simulink model "RadioReceiver_FP_clean_PIPELINED"  (R2017a)
settings: Solver=FixedStepDiscrete  StartTime=0.0  StopTime=10.0  RelTol=1e-3
InitFcn:
  | barker = comm.BarkerCode('SamplesPerFrame', 28, 'Length', 11);
  | seq = barker()+1;
  | M = 4;
  | hPSKModTrain   = comm.PSKModulator(M, ...
  |     'PhaseOffset',pi/4, ...
  |     'SymbolMapping','Binary');
  | xPreambleSeq = hPSKModTrain(seq);
  | 
  | 
  | %%%%%%%%%%%%
  | 
  | % AGC Preamble
  | reps = 5;
  | barker = comm.BarkerCode('SamplesPerFrame', 16, 'Length', 13);
  | seq = barker()+1;
  | %preamble = zeros(16*reps,1);
  | preambleFull = repmat(seq,reps,1);
  | rctFilt = comm.RaisedCosineTransmitFilter('FilterSpanInSymbols', 128,...
  | 'RolloffFactor',0.5,...
  | 'OutputSamplesPerSymbol',4);
  | preambleFullFilt = rctFilt(preambleFull);
  | 
  | %%%%%%%%%%%%
  | 
  | RadioSampleRate = 1e6;
  | %RadioSampleRate = 20e6;
  | RadioFrameLength = 1e5;
  | 
  | VibertiTracebackLength = 34+20;
  | numTrainingSamples = 250;
  | crc32Poly = [1 0 0 0 0 0 1 0 0 1 1 0 0 0 0 0 1 0 0 0 1 1 1 0 1 1 0 1 1 0 1 1 1];
  | crcDecodeLag = length(crc32Poly)-1+2;
  | 
  | %%%%%%%%%%%%
  | 
  | beta = 0.5;
  | span = 8;
  | sps = 4;
  | filterGain = 1;
  | coeff = rcosdesign(beta, span, sps, 'sqrt')*filterGain;
  | 
  | %%%%%%%%%%%%
  | 
  | samplesPerSymbol = 4;
  | maxPacketBits = 8*1500;
  | bItsPerSymbol = 2;
  | CodeRate = 2;
  | tailSymbols = 40;
  | maxPayloadSymbols = maxPacketBits*CodeRate/bItsPerSymbol+tailSymbols;
undefined symbols (not defined in the file or in its folder): j
libraries: dsphdlfiltering x20, simulink x11, dspstat3 x2, commdigbbndpm3 x2, commsource2 x1, commcrc2 x1, commcnvcod2 x1, commseqgen3 x1, commutil2 x1, hdlsllib x1
(part 1 of 2)
settings Model: DataTypeOverride=Off  MinMaxOverflowLogging=MinMaxAndOverflow  FPTRunName=NoOverride  Creator=tcollins  LastModifiedBy=tcollins
settings DataIOCC: SaveOutput=off  SaveTime=off
settings OptimizationCC: BlockReduction=off  ConditionallyExecuteInputs=off  DefaultParameterBehavior=Inlined
settings DebuggingCC: AlgebraicLoopMsg=error  SingleTaskRateTransMsg=error
settings HardwareCC: ProdBitPerPointer=32  ProdBitPerSizeT=32  ProdBitPerPtrDiffT=32  ProdLargestAtomicFloat=None  ProdIntDivRoundTo=Undefined  ProdEndianess=Unspecified  ProdWordSize=32  ProdHWDeviceType=ASIC/FPGA->ASIC/FPGA  ProdEqTarget=off

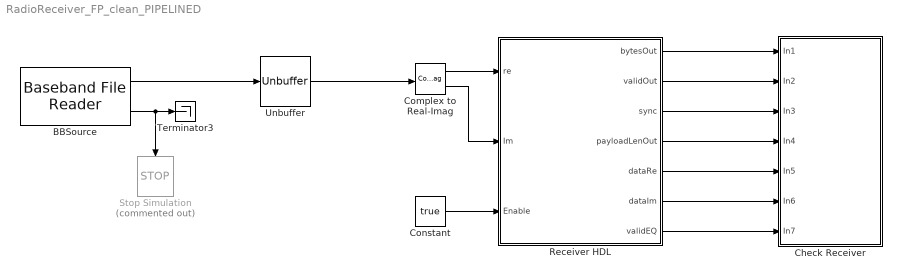
== system RadioReceiver_FP_clean_PIPELINED ==
  BBSource : commsource2/Baseband File Reader  Filename=/home/tcollins/currentWork/modem-phy/FixedPoint/Pluto3.bb  InheritSampleTimeFromFile=off  SampleTime=100000/(RadioSampleRate)  SamplesPerFrame=100000  CyclicRepetition=off  FileEndOutputPort=on  SimulateUsing=Interpreted execution
      settings: SourceProductName=Communications System Toolbox  SourceProductBaseCode=CM
  Check Receiver : Subsystem
  Complex to Real-Imag : ComplexToRealImag
  Constant : Constant  Value=true  SampleTime=1/RadioSampleRate
  Receiver HDL : Subsystem  TreatAsAtomicUnit=on
  Stop Simulation : Stop  Commented=on
  Terminator3 : Terminator
  Unbuffer : Unbuffer
  wires:
  BBSource/1 -> Unbuffer/1
  Constant/1 -> Receiver HDL/3(Enable)
  Complex to Real-Imag/1 -> Receiver HDL/1(re)
  Complex to Real-Imag/2 -> Receiver HDL/2(Im)
  BBSource/2 -> Stop Simulation/1, Terminator3/1
  Unbuffer/1 -> Complex to Real-Imag/1
  Receiver HDL/1(bytesOut) -> Check Receiver/1(In1)
  Receiver HDL/2(validOut) -> Check Receiver/2(In2)
  Receiver HDL/3(sync) -> Check Receiver/3(In3)
  Receiver HDL/4(payloadLenOut) -> Check Receiver/4(In4)
  Receiver HDL/5(dataRe) -> Check Receiver/5(In5)
  Receiver HDL/6(dataIm) -> Check Receiver/6(In6)
  Receiver HDL/7(validEQ) -> Check Receiver/7(In7)

== system RadioReceiver_FP_clean_PIPELINED/Check Receiver ==
  In1 : Inport
  In2 : Inport  Port=2
  In3 : Inport  Port=3
  In4 : Inport  Port=4
  In5 : Inport  Port=5
  In6 : Inport  Port=6
  In7 : Inport  Port=7
  Constellation Diagram : Subsystem
  DMA Capture : MATLAB Function  TreatAsAtomicUnit=on
  Real-Imag to Complex : RealImagToComplex
  wires:
  Real-Imag to Complex/1 -> Constellation Diagram/1(In1)
  In5/1 -> Real-Imag to Complex/1
  In3/1 -> DMA Capture/3(sync)
  In7/1 -> Constellation Diagram/Enable
  In2/1 -> DMA Capture/2(validOut)
  In1/1 -> DMA Capture/1(bytes)
  In4/1 -> DMA Capture/4(payloadLen)
  In6/1 -> Real-Imag to Complex/2

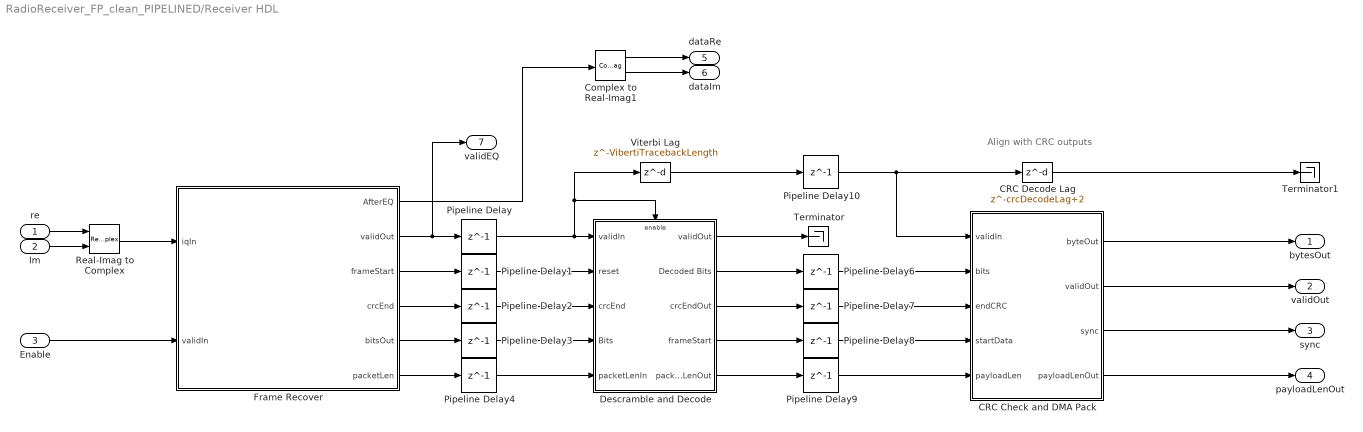
== system RadioReceiver_FP_clean_PIPELINED/Receiver HDL ==
  note: Align with CRC outputs
  re : Inport  OutDataTypeStr=int16
  Im : Inport  Port=2  OutDataTypeStr=int16
  Enable : Inport  Port=3
  CRC Check and DMA Pack : Subsystem
  CRC Decode Lag : Delay  DelayLength=crcDecodeLag+2
  Complex to Real-Imag1 : ComplexToRealImag
  Descramble and Decode : Subsystem  TreatAsAtomicUnit=on
  Frame Recover : Subsystem
  Pipeline Delay{,1..4,6..10} (10 alike) : Delay  DelayLength=1
  Real-Imag to Complex : RealImagToComplex
  Terminator : Terminator
  Terminator1 : Terminator
  Viterbi Lag : Delay  DelayLength=VibertiTracebackLength
  bytesOut : Outport
  validOut : Outport  Port=2
  sync : Outport  Port=3
  payloadLenOut : Outport  Port=4
  dataRe : Outport  Port=5
  dataIm : Outport  Port=6
  validEQ : Outport  Port=7
  wires:
  re/1 -> Real-Imag to Complex/1
  Im/1 -> Real-Imag to Complex/2
  Complex to Real-Imag1/2 -> dataIm/1
  Complex to Real-Imag1/1 -> dataRe/1
  Frame Recover/6(packetLen) -> Pipeline Delay4/1
  Frame Recover/2(validOut) -> validEQ/1, Pipeline Delay/1
  Real-Imag to Complex/1 -> Frame Recover/1(iqIn)
  Enable/1 -> Frame Recover/2(validIn)
  Frame Recover/1(AfterEQ) -> Complex to Real-Imag1/1
  Frame Recover/3(frameStart) -> Pipeline Delay1/1
  Frame Recover/4(crcEnd) -> Pipeline Delay2/1
  Frame Recover/5(bitsOut) -> Pipeline Delay3/1
  Descramble and Decode/3(crcEndOut) -> Pipeline Delay7/1
  Descramble and Decode/4(frameStart) -> Pipeline Delay8/1
  Descramble and Decode/5(packetLenOut) -> Pipeline Delay9/1
  CRC Check and DMA Pack/1(byteOut) -> bytesOut/1
  CRC Check and DMA Pack/2(validOut) -> validOut/1
  Pipeline Delay1/1 -> Descramble and Decode/2(reset)
  Pipeline Delay3/1 -> Descramble and Decode/4(Bits)
  Pipeline Delay4/1 -> Descramble and Decode/5(packetLenIn)
  Pipeline Delay8/1 -> CRC Check and DMA Pack/4(startData)
  Pipeline Delay6/1 -> CRC Check and DMA Pack/2(bits)
  Pipeline Delay9/1 -> CRC Check and DMA Pack/5(payloadLen)
  Pipeline Delay7/1 -> CRC Check and DMA Pack/3(endCRC)
  CRC Check and DMA Pack/3(sync) -> sync/1
  Pipeline Delay2/1 -> Descramble and Decode/3(crcEnd)
  Descramble and Decode/2(Decoded Bits) -> Pipeline Delay6/1
  Pipeline Delay10/1 -> CRC Check and DMA Pack/1(validIn), CRC Decode Lag/1
  CRC Check and DMA Pack/4(payloadLenOut) -> payloadLenOut/1
  Pipeline Delay/1 -> Descramble and Decode/Enable, Viterbi Lag/1, Descramble and Decode/1(validIn)
  Descramble and Decode/1(validOut) -> Terminator/1
  Viterbi Lag/1 -> Pipeline Delay10/1
  CRC Decode Lag/1 -> Terminator1/1

== system RadioReceiver_FP_clean_PIPELINED/Check Receiver/Constellation Diagram ==
  In1 : Inport
  Enable : EnablePort
  After EQ (Outside) : ConstellationDiagram
  wires:
  In1/1 -> After EQ (Outside)/1

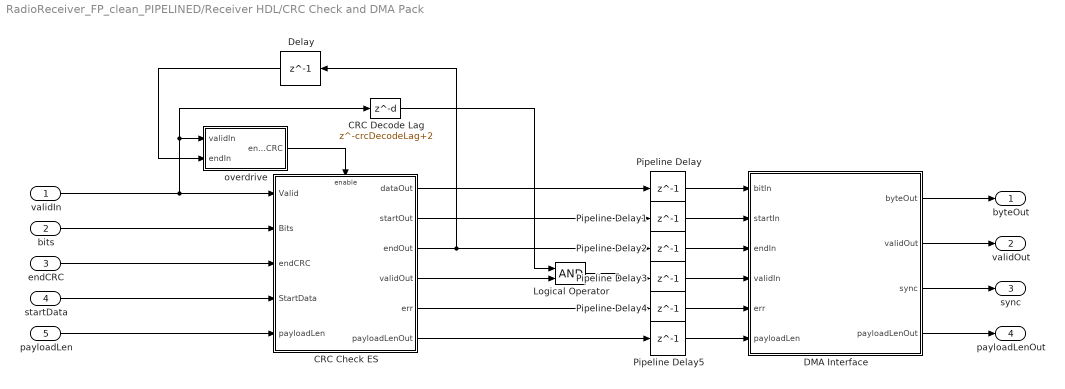
== system RadioReceiver_FP_clean_PIPELINED/Receiver HDL/CRC Check and DMA Pack ==
  validIn : Inport
  bits : Inport  Port=2
  endCRC : Inport  Port=3
  startData : Inport  Port=4
  payloadLen : Inport  Port=5
  CRC Check ES : Subsystem
  CRC Decode Lag : Delay  DelayLength=crcDecodeLag+2
  DMA Interface : Subsystem
  Delay : Delay  DelayLength=1
  Logical Operator : Logic  AllPortsSameDT=off  OutDataTypeStr=boolean
  Pipeline Delay{,1..5} (6 alike) : Delay  DelayLength=1
  overdrive : MATLAB Function  TreatAsAtomicUnit=on
  byteOut : Outport
  validOut : Outport  Port=2
  sync : Outport  Port=3
  payloadLenOut : Outport  Port=4
  wires:
  DMA Interface/2(validOut) -> validOut/1
  CRC Check ES/3(endOut) -> Delay/1, Pipeline Delay2/1
  DMA Interface/1(byteOut) -> byteOut/1
  CRC Check ES/2(startOut) -> Pipeline Delay1/1
  CRC Check ES/1(dataOut) -> Pipeline Delay/1
  CRC Check ES/5(err) -> Pipeline Delay4/1
  bits/1 -> CRC Check ES/2(Bits)
  DMA Interface/3(sync) -> sync/1
  payloadLen/1 -> CRC Check ES/5(payloadLen)
  startData/1 -> CRC Check ES/4(StartData)
  CRC Check ES/6(payloadLenOut) -> Pipeline Delay5/1
  endCRC/1 -> CRC Check ES/3(endCRC)
  Pipeline Delay/1 -> DMA Interface/1(bitIn)
  Pipeline Delay1/1 -> DMA Interface/2(startIn)
  Pipeline Delay2/1 -> DMA Interface/3(endIn)
  Pipeline Delay3/1 -> DMA Interface/4(validIn)
  Pipeline Delay4/1 -> DMA Interface/5(err)
  Pipeline Delay5/1 -> DMA Interface/6(payloadLen)
  CRC Decode Lag/1 -> Logical Operator/1
  CRC Check ES/4(validOut) -> Logical Operator/2
  validIn/1 -> CRC Check ES/1(Valid), CRC Decode Lag/1, overdrive/1(validIn)
  Delay/1 -> overdrive/2(endIn)
  DMA Interface/4(payloadLenOut) -> payloadLenOut/1
  Logical Operator/1 -> Pipeline Delay3/1
  overdrive/1(enableCRC) -> CRC Check ES/Enable

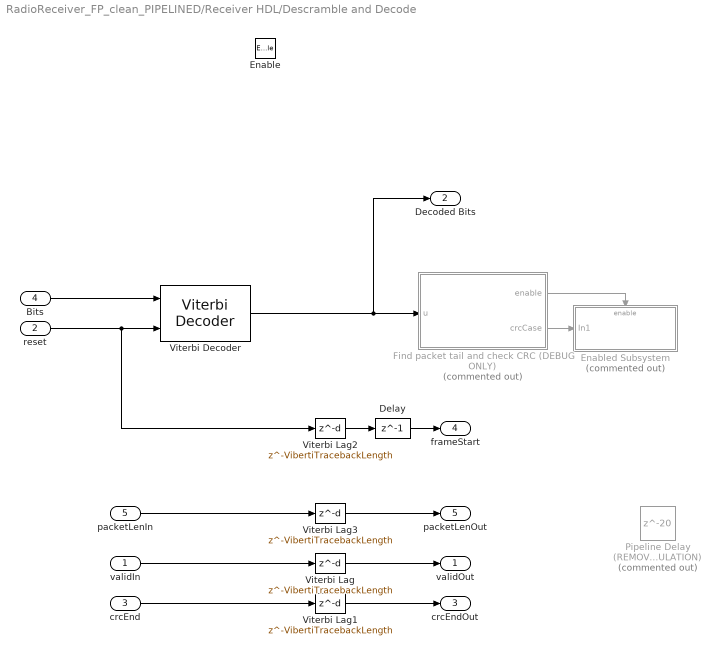
== system RadioReceiver_FP_clean_PIPELINED/Receiver HDL/Descramble and Decode ==
  validIn : Inport
  reset : Inport  Port=2
  crcEnd : Inport  Port=3
  Bits : Inport  Port=4
  packetLenIn : Inport  Port=5
  Enable : EnablePort
  Delay : Delay  DelayLength=1
  Enabled Subsystem : Subsystem  Commented=on  TreatAsAtomicUnit=on
  Find packet tail and check CRC (DEBUG ONLY) : MATLAB Function  Commented=on  TreatAsAtomicUnit=on
  "Pipeline Delay (REMOVE BEFORE SYNTH, ONLY FOR SIMULATION)" : Delay  Commented=on  DelayLength=20
  Viterbi Decoder : commcnvcod2/Viterbi Decoder  trellis=poly2trellis(7, [171 133])  isPunctured=off  punctureVector=[1; 1; 0; 1; 0; 1]  erasures=off  dectype=Hard decision  nsdecb=4  runSigValErrCheck=off  tbdepth=VibertiTracebackLength-20  opmode=Continuous  reset=on  delayedResetAction=on  smWordLength=16  outDataType=boolean
      settings: SourceProductName=Communications System Toolbox  SourceProductBaseCode=CM
  Viterbi Lag{,1..3} (4 alike) : Delay  DelayLength=VibertiTracebackLength
  validOut : Outport  InitialOutput=0
  Decoded Bits : Outport  Port=2  InitialOutput=0
  crcEndOut : Outport  Port=3  InitialOutput=0
  frameStart : Outport  Port=4  InitialOutput=0
  packetLenOut : Outport  Port=5  InitialOutput=0
  wires:
  reset/1 -> Viterbi Lag2/1, Viterbi Decoder/2
  Find packet tail and check CRC (DEBUG ONLY)/1(enable) -> Enabled Subsystem/Enable
  Find packet tail and check CRC (DEBUG ONLY)/2(crcCase) -> Enabled Subsystem/1(In1)
  Bits/1 -> Viterbi Decoder/1
  validIn/1 -> Viterbi Lag/1
  Viterbi Lag3/1 -> packetLenOut/1
  Viterbi Lag2/1 -> Delay/1
  Viterbi Lag1/1 -> crcEndOut/1
  Viterbi Lag/1 -> validOut/1
  packetLenIn/1 -> Viterbi Lag3/1
  crcEnd/1 -> Viterbi Lag1/1
  Delay/1 -> frameStart/1
  Viterbi Decoder/1 -> Decoded Bits/1, Find packet tail and check CRC (DEBUG ONLY)/1(u)

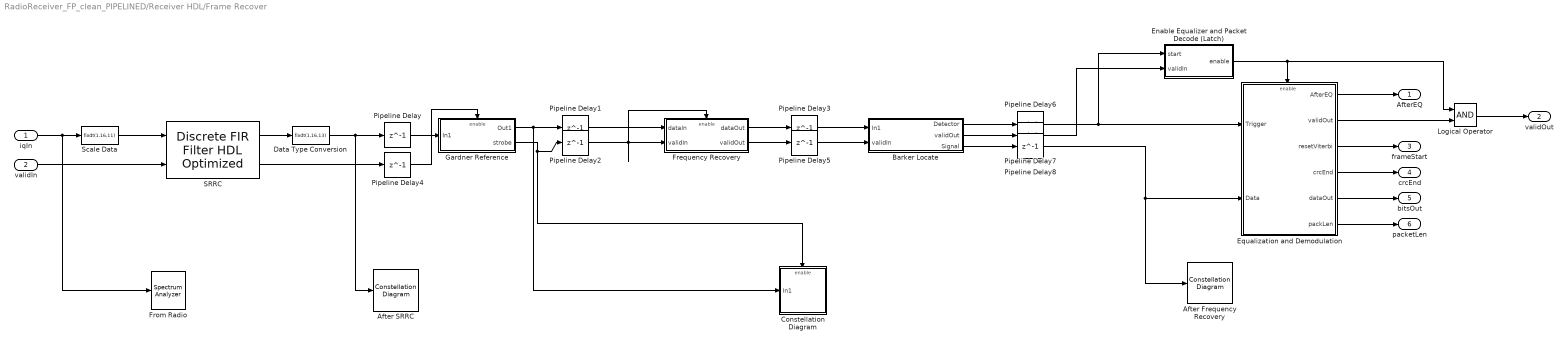
== system RadioReceiver_FP_clean_PIPELINED/Receiver HDL/Frame Recover ==
  iqIn : Inport
  validIn : Inport  Port=2
  After Frequency Recovery : ConstellationDiagram
  After SRRC : ConstellationDiagram
  Barker Locate : Subsystem  mask{Threshold=1}
  Constellation Diagram : Subsystem
  Data Type Conversion : DataTypeConversion  OutDataTypeStr=fixdt(1,16,13)
  Enable Equalizer and Packet Decode (Latch) : MATLAB Function  TreatAsAtomicUnit=on
  Equalization and Demodulation : Subsystem
  Frequency Recovery : Subsystem
  From Radio : SpectrumAnalyzer
  Gardner Reference : Subsystem
  Logical Operator : Logic  AllPortsSameDT=off  OutDataTypeStr=boolean
  Pipeline Delay{,1..8} (9 alike) : Delay  DelayLength=1
  SRRC : dsphdlfiltering/Discrete FIR Filter HDL Optimized  Numerator=coeff  Sharing=off  SharingFactor=2  SimulateUsing=Code generation  roundingMode=Floor  overflowMode=on  CoefficientsDataTypeStr=Inherit: Same word length as input  CoefficientsMin=[]  CoefficientsMax=[]  OutputDataTypeStr=fixdt(1,16,11)  OutputMin=[]  OutputMax=[]  ValidInPort=on  ReadyPort=off
      settings: SourceProductName=DSP System Toolbox  SourceProductBaseCode=DS
  Scale Data : DataTypeConversion  OutDataTypeStr=fixdt(1,16,11)  ConvertRealWorld=Stored Integer (SI)  SaturateOnIntegerOverflow=on
  AfterEQ : Outport
  validOut : Outport  Port=2
  frameStart : Outport  Port=3
  crcEnd : Outport  Port=4
  bitsOut : Outport  Port=5
  packetLen : Outport  Port=6
  wires:
  Equalization and Demodulation/3(resetViterbi) -> frameStart/1
  Barker Locate/2(validOut) -> Pipeline Delay7/1
  Equalization and Demodulation/4(crcEnd) -> crcEnd/1
  Frequency Recovery/2(validOut) -> Pipeline Delay5/1
  Enable Equalizer and Packet Decode (Latch)/1(enable) -> Logical Operator/1, Equalization and Demodulation/Enable
  Equalization and Demodulation/5(dataOut) -> bitsOut/1
  SRRC/2 -> Pipeline Delay4/1
  SRRC/1 -> Data Type Conversion/1
  iqIn/1 -> From Radio/1, Scale Data/1
  validIn/1 -> SRRC/2
  Barker Locate/3(Signal) -> Pipeline Delay8/1
  Frequency Recovery/1(dataOut) -> Pipeline Delay3/1
  Equalization and Demodulation/2(validOut) -> Logical Operator/2
  Scale Data/1 -> SRRC/1
  Equalization and Demodulation/6(packLen) -> packetLen/1
  Barker Locate/1(Detector) -> Pipeline Delay6/1
  Equalization and Demodulation/1(AfterEQ) -> AfterEQ/1
  Pipeline Delay1/1 -> Frequency Recovery/1(dataIn)
  Pipeline Delay2/1 -> Frequency Recovery/Enable, Frequency Recovery/2(validIn)
  Pipeline Delay3/1 -> Barker Locate/1(In1)
  Pipeline Delay5/1 -> Barker Locate/2(validIn)
  Pipeline Delay6/1 -> Enable Equalizer and Packet Decode (Latch)/1(start), Equalization and Demodulation/1(Trigger)
  Pipeline Delay7/1 -> Enable Equalizer and Packet Decode (Latch)/2(validIn)
  Pipeline Delay8/1 -> Equalization and Demodulation/2(Data), After Frequency Recovery/1
  Logical Operator/1 -> validOut/1
  Data Type Conversion/1 -> After SRRC/1, Pipeline Delay/1
  Pipeline Delay/1 -> Gardner Reference/1(In1)
  Gardner Reference/2(strobe) -> Pipeline Delay2/1, Constellation Diagram/Enable
  Gardner Reference/1(Out1) -> Constellation Diagram/1(In1), Pipeline Delay1/1
  Pipeline Delay4/1 -> Gardner Reference/Enable

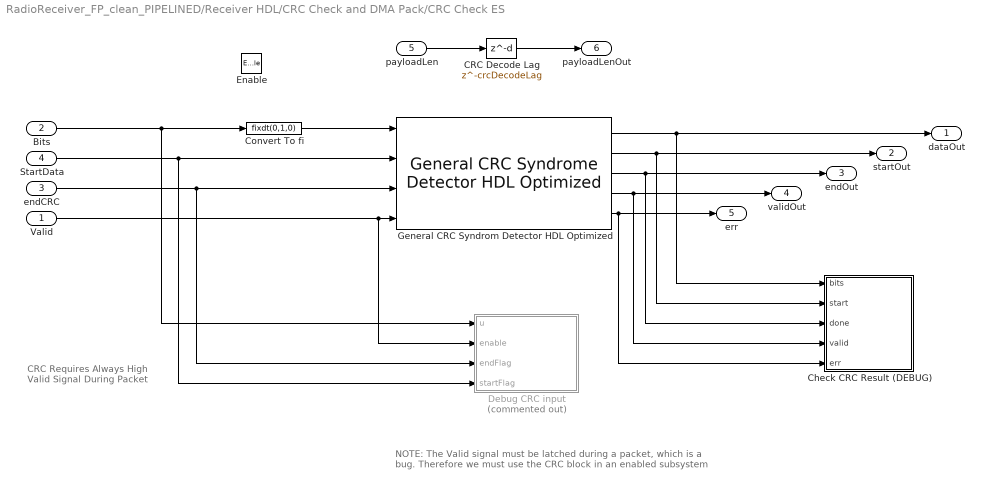
== system RadioReceiver_FP_clean_PIPELINED/Receiver HDL/CRC Check and DMA Pack/CRC Check ES ==
  note: NOTE:
      | 	The Valid signal must be latched during a packet, which is
      | 	a bug.  Therefore we must use the CRC block in an enabled
      | 	subsystem
  note: CRC Requires
      | Always High
      | Valid Signal During
      | Packet
  Valid : Inport
  Bits : Inport  Port=2
  endCRC : Inport  Port=3
  StartData : Inport  Port=4
  payloadLen : Inport  Port=5
  Enable : EnablePort
  CRC Decode Lag : Delay  DelayLength=crcDecodeLag
  Check CRC Result (DEBUG) : MATLAB Function  TreatAsAtomicUnit=on
  Convert To fi : DataTypeConversion  OutDataTypeStr=fixdt(0,1,0)  SaturateOnIntegerOverflow=on
  Debug CRC input : MATLAB Function  Commented=on  TreatAsAtomicUnit=on
  General CRC Syndrom Detector HDL Optimized : commcrc2/General CRC Syndrome Detector HDL Optimized  Polynomial=crc32Poly  InitialState=0  DirectMethod=off  ReflectInput=off  ReflectCRCChecksum=off  FinalXORValue=0  SimulateUsing=Code generation
      settings: SourceProductName=Communications System Toolbox  SourceProductBaseCode=CM
  dataOut : Outport  InitialOutput=0
  startOut : Outport  Port=2  InitialOutput=0
  endOut : Outport  Port=3  InitialOutput=0
  validOut : Outport  Port=4  InitialOutput=0
  err : Outport  Port=5  InitialOutput=0
  payloadLenOut : Outport  Port=6  InitialOutput=0
  wires:
  Bits/1 -> Convert To fi/1, Debug CRC input/1(u)
  General CRC Syndrom Detector HDL Optimized/1 -> Check CRC Result (DEBUG)/1(bits), dataOut/1
  General CRC Syndrom Detector HDL Optimized/3 -> Check CRC Result (DEBUG)/3(done), endOut/1
  General CRC Syndrom Detector HDL Optimized/4 -> Check CRC Result (DEBUG)/4(valid), validOut/1
  General CRC Syndrom Detector HDL Optimized/5 -> Check CRC Result (DEBUG)/5(err), err/1
  General CRC Syndrom Detector HDL Optimized/2 -> Check CRC Result (DEBUG)/2(start), startOut/1
  Convert To fi/1 -> General CRC Syndrom Detector HDL Optimized/1
  payloadLen/1 -> CRC Decode Lag/1
  CRC Decode Lag/1 -> payloadLenOut/1
  StartData/1 -> Debug CRC input/4(startFlag), General CRC Syndrom Detector HDL Optimized/2
  endCRC/1 -> Debug CRC input/3(endFlag), General CRC Syndrom Detector HDL Optimized/3
  Valid/1 -> Debug CRC input/2(enable), General CRC Syndrom Detector HDL Optimized/4

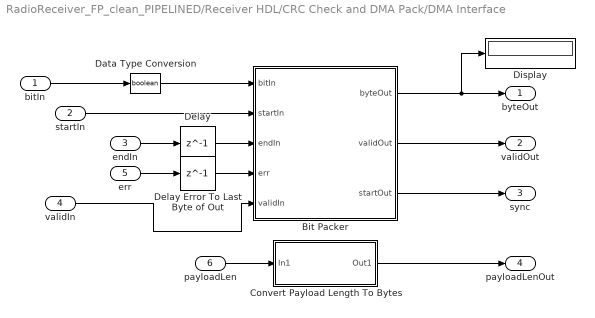
== system RadioReceiver_FP_clean_PIPELINED/Receiver HDL/CRC Check and DMA Pack/DMA Interface ==
  bitIn : Inport
  startIn : Inport  Port=2
  endIn : Inport  Port=3
  validIn : Inport  Port=4
  err : Inport  Port=5
  payloadLen : Inport  Port=6
  Bit Packer : MATLAB Function  TreatAsAtomicUnit=on
  Convert Payload Length To Bytes : Subsystem
  Data Type Conversion : DataTypeConversion  OutDataTypeStr=boolean
  Delay : Delay  DelayLength=1
  Delay Error To Last Byte of Out : Delay  DelayLength=1
  Display : Display
  byteOut : Outport
  validOut : Outport  Port=2
  sync : Outport  Port=3
  payloadLenOut : Outport  Port=4
  wires:
  bitIn/1 -> Data Type Conversion/1
  Delay/1 -> Bit Packer/3(endIn)
  Delay Error To Last Byte of Out/1 -> Bit Packer/4(err)
  Bit Packer/2(validOut) -> validOut/1
  Bit Packer/3(startOut) -> sync/1
  Bit Packer/1(byteOut) -> Display/1, byteOut/1
  err/1 -> Delay Error To Last Byte of Out/1
  validIn/1 -> Bit Packer/5(validIn)
  endIn/1 -> Delay/1
  startIn/1 -> Bit Packer/2(startIn)
  Data Type Conversion/1 -> Bit Packer/1(bitIn)
  payloadLen/1 -> Convert Payload Length To Bytes/1(In1)
  Convert Payload Length To Bytes/1(Out1) -> payloadLenOut/1

== system RadioReceiver_FP_clean_PIPELINED/Receiver HDL/Descramble and Decode/Enabled Subsystem ==
  In1 : Inport
  Enable : EnablePort
  To Workspace : ToWorkspace  VariableName=crcConditions  SaveFormat=Structure  SampleTime=-1
  wires:
  In1/1 -> To Workspace/1

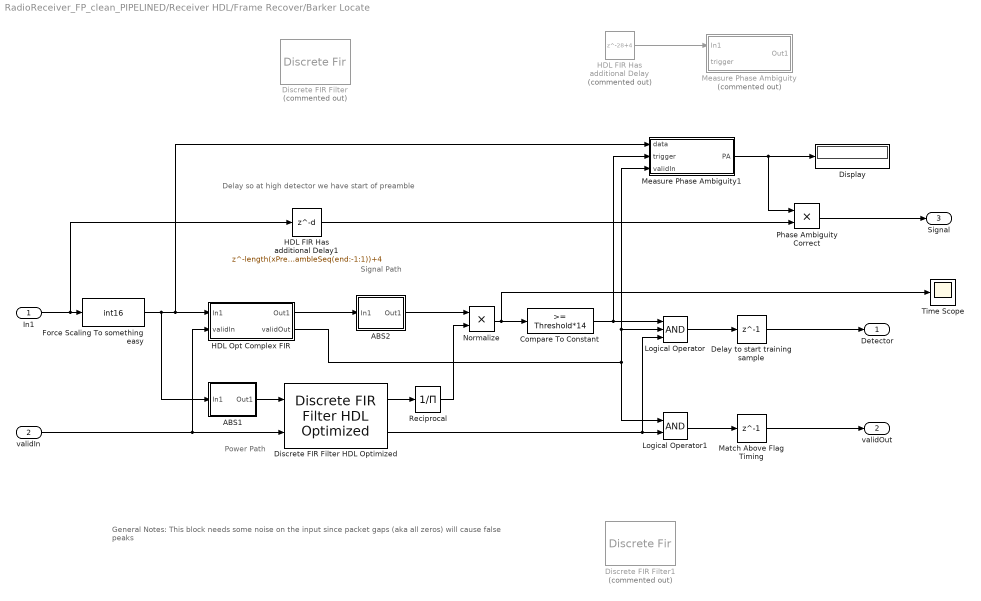
== system RadioReceiver_FP_clean_PIPELINED/Receiver HDL/Frame Recover/Barker Locate ==
  note: General Notes:
      | This block needs some noise on the input since packet gaps (aka all zeros) will cause false peaks
  note: Delay so at high detector we have start of preamble
  note: Power Path
  note: Signal Path
  In1 : Inport
  validIn : Inport  Port=2
  ABS1 : Subsystem
  ABS2 : Subsystem
  Compare To Constant : simulink/Logic and Bit Operations/Compare To Constant  relop=>=  const=Threshold*14  OutDataTypeStr=boolean
  "Delay to start training sample " : Delay  DelayLength=1
  Discrete FIR Filter : DiscreteFir  Commented=on  Coefficients=xPreambleSeq(end:-1:1).'  AccumDataTypeStr=Inherit: Same as product output  OutDataTypeStr=int16
  Discrete FIR Filter HDL Optimized : dsphdlfiltering/Discrete FIR Filter HDL Optimized  Numerator=ones(1,length(xPreambleSeq)*1)/1  Sharing=off  SharingFactor=2  SimulateUsing=Code generation  roundingMode=Floor  overflowMode=off  CoefficientsDataTypeStr=Inherit: Same word length as input  CoefficientsMin=[]  CoefficientsMax=[]  OutputDataTypeStr=fixdt(1,17,0)  OutputMin=[]  OutputMax=[]  ValidInPort=on  ReadyPort=off
      settings: SourceProductName=DSP System Toolbox  SourceProductBaseCode=DS
  Discrete FIR Filter1 : DiscreteFir  Commented=on  Coefficients=ones(1,length(xPreambleSeq)*1)/1  AccumDataTypeStr=Inherit: Same as product output  OutDataTypeStr=int16  SaturateOnIntegerOverflow=on
  Display : Display
  Force Scaling To something easy : DataTypeConversion  OutDataTypeStr=int16  SaturateOnIntegerOverflow=on
  HDL FIR Has additional Delay : Delay  Commented=on  DelayLength=28+4
  HDL FIR Has additional Delay1 : Delay  DelayLength=length(xPreambleSeq(end:-1:1))+4
  HDL Opt Complex FIR : Subsystem  mask{Taps=xPreambleSeq(end:-1:1).'}
  Logical Operator : Logic  Inputs=3  AllPortsSameDT=off  OutDataTypeStr=boolean
  Logical Operator1 : Logic  AllPortsSameDT=off  OutDataTypeStr=boolean
  Match Above Flag Timing : Delay  DelayLength=1
  Measure Phase Ambiguity : Subsystem  Commented=on
  Measure Phase Ambiguity1 : Subsystem
  Normalize : Product  Inputs=**  OutDataTypeStr=int16  RndMeth=Simplest  SaturateOnIntegerOverflow=on
  Phase Ambiguity Correct : Product  OutDataTypeStr=fixdt(1,16,14)
  Reciprocal : Product  Inputs=/  SaturateOnIntegerOverflow=on  RndMeth=Zero
  Time Scope : Scope
  Detector : Outport
  validOut : Outport  Port=2
  Signal : Outport  Port=3
  wires:
  HDL Opt Complex FIR/1(Out1) -> ABS2/1(In1)
  ABS2/1(Out1) -> Normalize/1
  "Delay to start training sample "/1 -> Detector/1
  Normalize/1 -> Time Scope/1, Compare To Constant/1
  In1/1 -> HDL FIR Has additional Delay1/1, Force Scaling To something easy/1
  ABS1/1(Out1) -> Discrete FIR Filter HDL Optimized/1
  Logical Operator/1 -> "Delay to start training sample "/1
  Logical Operator1/1 -> Match Above Flag Timing/1
  Measure Phase Ambiguity1/1(PA) -> Display/1, Phase Ambiguity Correct/1
  validIn/1 -> HDL Opt Complex FIR/2(validIn), Discrete FIR Filter HDL Optimized/2
  Discrete FIR Filter HDL Optimized/2 -> Logical Operator1/2, Logical Operator/3
  HDL Opt Complex FIR/2(validOut) -> Logical Operator1/1, Measure Phase Ambiguity1/3(validIn), Logical Operator/2
  Phase Ambiguity Correct/1 -> Signal/1
  HDL FIR Has additional Delay1/1 -> Phase Ambiguity Correct/2
  Force Scaling To something easy/1 -> ABS1/1(In1), HDL Opt Complex FIR/1(In1), Measure Phase Ambiguity1/1(data)
  Compare To Constant/1 -> Measure Phase Ambiguity1/2(trigger), Logical Operator/1
  HDL FIR Has additional Delay/1 -> Measure Phase Ambiguity/1(In1)
  Discrete FIR Filter HDL Optimized/1 -> Reciprocal/1
  Reciprocal/1 -> Normalize/2
  Match Above Flag Timing/1 -> validOut/1

== system RadioReceiver_FP_clean_PIPELINED/Receiver HDL/Frame Recover/Constellation Diagram ==
  In1 : Inport
  Enable : EnablePort
  After Timing Recovery : ConstellationDiagram
  wires:
  In1/1 -> After Timing Recovery/1

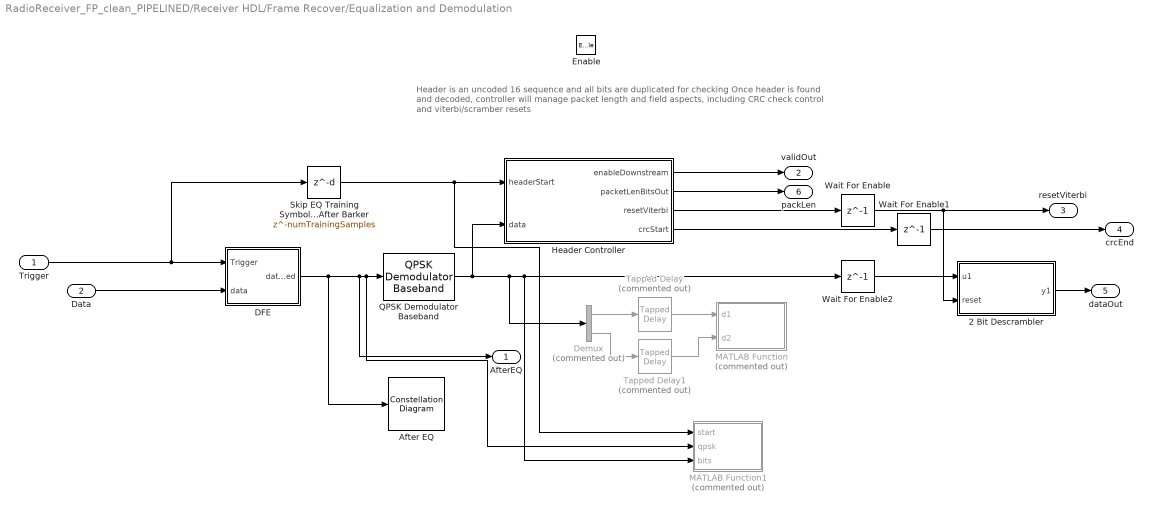
== system RadioReceiver_FP_clean_PIPELINED/Receiver HDL/Frame Recover/Equalization and Demodulation ==
  note: Header is an uncoded 16 sequence and all bits are duplicated for checking
      |
      | Once header is found and decoded, controller will manage packet length and field aspects,
      | including CRC check control and viterbi/scramber resets
  Trigger : Inport
  Data : Inport  Port=2
  Enable : EnablePort
  2 Bit Descrambler : Subsystem  mask{polynom=[1 1 0 1 0 1 0 1], initstate=[0 1 0 0 0 1 0]}
      mask prompts: polynom "Polynomial"; initstate "Inital State"
      mask Display: fprintf('HDL Descrambler')
  After EQ : ConstellationDiagram
  DFE : Subsystem
  Demux : Demux  Commented=on  Outputs=2
  Header Controller : MATLAB Function  TreatAsAtomicUnit=on
  MATLAB Function : MATLAB Function  Commented=on  TreatAsAtomicUnit=on
  MATLAB Function1 : MATLAB Function  Commented=on  TreatAsAtomicUnit=on
  QPSK Demodulator Baseband : commdigbbndpm3/QPSK Demodulator Baseband  OutType=Bit  DecType=Hard decision  VarSource=Dialog  Variance=1  Dec=Binary  Ph=pi/4  outDtype1=boolean  outDtype2=Inherit via internal rule  derotateFactorWordLen=16  derotateFactorDataTypeStr=Inherit: Same word length as input  derotateFactorLastDataTypeStr=Inherit: Same word length as input
  Skip EQ Training Symbols After Barker : Delay  DelayLength=numTrainingSamples
  Tapped Delay : simulink/Discrete/Tapped Delay  Commented=on  vinit=0.0  samptime=-1  NumDelays=16  DelayOrder=Oldest  includeCurrent=off
  Tapped Delay1 : simulink/Discrete/Tapped Delay  Commented=on  vinit=0.0  samptime=-1  NumDelays=16  DelayOrder=Oldest  includeCurrent=off
  Wait For Enable : Delay  DelayLength=1
  Wait For Enable1 : Delay  DelayLength=1
  Wait For Enable2 : Delay  DelayLength=1
  AfterEQ : Outport  InitialOutput=0
  validOut : Outport  Port=2  InitialOutput=0
  resetViterbi : Outport  Port=3  InitialOutput=0
  crcEnd : Outport  Port=4  InitialOutput=0
  dataOut : Outport  Port=5  InitialOutput=0
  packLen : Outport  Port=6  InitialOutput=0
  wires:
  Skip EQ Training Symbols After Barker/1 -> MATLAB Function1/1(start), Header Controller/1(headerStart)
  DFE/1(dataEQed) -> AfterEQ/1, MATLAB Function1/2(qpsk), QPSK Demodulator Baseband/1, After EQ/1
  QPSK Demodulator Baseband/1 -> Header Controller/2(data), Demux/1, MATLAB Function1/3(bits), Wait For Enable2/1
  Header Controller/1(enableDownstream) -> validOut/1
  Header Controller/4(crcStart) -> Wait For Enable1/1
  Header Controller/3(resetViterbi) -> Wait For Enable/1
  Header Controller/2(packetLenBitsOut) -> packLen/1
  Wait For Enable/1 -> 2 Bit Descrambler/2(reset), resetViterbi/1
  Wait For Enable1/1 -> crcEnd/1
  Wait For Enable2/1 -> 2 Bit Descrambler/1(u1)
  2 Bit Descrambler/1(y1) -> dataOut/1
  Demux/1 -> Tapped Delay/1
  Demux/2 -> Tapped Delay1/1
  Tapped Delay/1 -> MATLAB Function/1(d1)
  Tapped Delay1/1 -> MATLAB Function/2(d2)
  Trigger/1 -> DFE/1(Trigger), Skip EQ Training Symbols After Barker/1
  Data/1 -> DFE/2(data)

== system RadioReceiver_FP_clean_PIPELINED/Receiver HDL/Frame Recover/Frequency Recovery ==
  note: Decrease Loop bandwidth to reduce phase noise,
      | but worse pull-in range
      | -0.1 30kHz pull-in
      | -0.01 5kHz pull-in
  note: Max Phase Lock Delay= 1.3/(NormLoopBandwidth*SampleRate)
  note: Frequency Lock Delay = SampleRate*4*NormalizedPullInRange^2)/ (SampleRate*NormLoopBandwidth)^3;
  note: Pull in range (Hz) = 2*pi*sqrt(2)*DampingFactor*NormLoopBandwidth*SampleRate
  dataIn : Inport
  validIn : Inport  Port=2
  Enable : EnablePort
  Data Type Conversion : DataTypeConversion  Commented=on  OutDataTypeStr=fixdt(1,16,10)
  Delay : Delay  DelayLength=1
  Loop Filter : Subsystem  mask{BnTs=0.01, zeta=4*1/sqrt(2), N=1}
      mask prompts: BnTs "Normalized Loop Bandwidth"; zeta "Damping Factor"; N "Number of Samples/Symbol"
      mask init:
      | % See C.57 to C.61 in Michael Rice's "Digital Communications 
      | % - A Discrete-Time Approach" for details
      | 
      | %theta = BnTs/(zeta+0.25/zeta);  %0.0385
      | %d = 1 + 2*zeta*theta + theta*theta; %1.1938
      | %K1 = zeta*theta/d; %0.0805
      | %K2 = theta*theta/(d*2); %6.1958e-04
      | 
      | %%
      | DampingFactor = zeta;
      | samplesPerSymbol = N;
      | NormalizedLoopBandwidth = BnTs;
      | %
      | PhaseRecoveryLoopBandwidth = NormalizedLoopBandwidth*samplesPerSymbol;
      |  
      | PhaseRecoveryGain = samplesPerSymbol;
      |  
      | PhaseErrorDetectorGain = 1;
      | 
      | 
      | theta = PhaseRecoveryLoopBandwidth/...
      |     ((DampingFactor + 0.25/DampingFactor)*samplesPerSymbol);
      |  
      | d = 1 + 2*DampingFactor*theta + theta*theta;
      |  
      | % K1
      | K1 = (4*DampingFactor*theta/d)/...
      |     (PhaseErrorDetectorGain*PhaseRecoveryGain);
      | % K2
      | K2 = (4/samplesPerSymbol*theta*theta/d)/...
      |     (PhaseErrorDetectorGain*PhaseRecoveryGain);
      mask Display: disp('Loop Filter')
  PED : MATLAB Function  TreatAsAtomicUnit=on
  PED For QPSK : Subsystem  Commented=on
  PED For QPSK1 : Subsystem  Commented=on
  Phase Shift FP : Subsystem
  State Control : StateControl  StateControl=Synchronous
  dataOut : Outport
  validOut : Outport  Port=2
  wires:
  Delay/1 -> PED/1(In), dataOut/1
  PED/1(e) -> Loop Filter/1(e)
  Loop Filter/1(v) -> Phase Shift FP/2(Phi)
  dataIn/1 -> Phase Shift FP/1(In1)
  Phase Shift FP/1(Out1) -> Delay/1
  validIn/1 -> validOut/1

== system RadioReceiver_FP_clean_PIPELINED/Receiver HDL/Frame Recover/Gardner Reference ==
  In1 : Inport
  Enable : EnablePort
  Delay : Delay  DelayLength=1
  Delay1 : Delay  DelayLength=1
  Delay2 : Delay  DelayLength=6
  Gardner TED Blocks : Subsystem
  InterpControl_Blocks1 : Subsystem
  Interpolator : Subsystem
  LoopFilter1 : Subsystem  mask{zeta=sqrt(2), BnTs=0.01, Kp=2.7}
      mask prompts: zeta "DampingFactor"; BnTs "NormalizedLoopBandwidth"; Kp "DetectionGain"
      mask init:
      | K0 = -1;
      | SPS = 4;
      | theta = BnTs/SPS/(zeta + 0.25/zeta);
      | d  = (1 + 2*zeta*theta + theta^2) * K0 * Kp;
      | ProportionalGain = (4*zeta*theta) /d;
      | IntegratorGain   = (4*theta*theta)/d;
  State Control : StateControl  StateControl=Synchronous
  Out1 : Outport  InitialOutput=0
  strobe : Outport  Port=2  InitialOutput=false
  wires:
  In1/1 -> Delay2/1
  Delay1/1 -> Gardner TED Blocks/2(strobe), strobe/1
  Delay/1 -> Interpolator/2(mu)
  Interpolator/1(Out1) -> Gardner TED Blocks/1(data), Out1/1
  Gardner TED Blocks/1(e) -> LoopFilter1/1(e)
  InterpControl_Blocks1/1(strobe) -> Delay1/1
  InterpControl_Blocks1/2(mu) -> Delay/1
  LoopFilter1/1(v) -> InterpControl_Blocks1/1(e)
  Delay2/1 -> Interpolator/1(In1)

== system RadioReceiver_FP_clean_PIPELINED/Receiver HDL/CRC Check and DMA Pack/DMA Interface/Convert Payload Length To Bytes ==
  In1 : Inport
  Constant : Constant  Value=uint16(32-1)  SampleTime=-1
  Convert To Bytes From Bits : ArithShift  BitShiftNumber=3  BitShiftDirection=Right
  Convert To Uncoded : ArithShift  BitShiftNumber=1  BitShiftDirection=Right
  Data Type Conversion : DataTypeConversion  OutDataTypeStr=uint32
  Remove CRC Length : Sum  Inputs=+-  AccumDataTypeStr=uint16
  Out1 : Outport
  wires:
  In1/1 -> Convert To Uncoded/1
  Remove CRC Length/1 -> Convert To Bytes From Bits/1
  Convert To Uncoded/1 -> Remove CRC Length/1
  Convert To Bytes From Bits/1 -> Data Type Conversion/1
  Constant/1 -> Remove CRC Length/2
  Data Type Conversion/1 -> Out1/1

== system RadioReceiver_FP_clean_PIPELINED/Receiver HDL/Frame Recover/Barker Locate/ABS1 ==
  In1 : Inport
  Add : Sum
  Complex to Real-Imag : ComplexToRealImag
  Product : Product  OutDataTypeStr=int16
  Product1 : Product  OutDataTypeStr=int16
  Out1 : Outport
  wires:
  In1/1 -> Complex to Real-Imag/1
  Complex to Real-Imag/2 -> Product1/2, Product1/1
  Complex to Real-Imag/1 -> Product/1, Product/2
  Product/1 -> Add/1
  Product1/1 -> Add/2
  Add/1 -> Out1/1

== system RadioReceiver_FP_clean_PIPELINED/Receiver HDL/Frame Recover/Barker Locate/ABS2 ==
  In1 : Inport
  Add : Sum  SaturateOnIntegerOverflow=on
  Complex to Real-Imag : ComplexToRealImag
  Product : Product  OutDataTypeStr=int16
  Product1 : Product  OutDataTypeStr=int16
  Out1 : Outport
  wires:
  In1/1 -> Complex to Real-Imag/1
  Complex to Real-Imag/2 -> Product1/2, Product1/1
  Complex to Real-Imag/1 -> Product/1, Product/2
  Product/1 -> Add/1
  Product1/1 -> Add/2
  Add/1 -> Out1/1

== system RadioReceiver_FP_clean_PIPELINED/Receiver HDL/Frame Recover/Barker Locate/HDL Opt Complex FIR ==
  In1 : Inport
  validIn : Inport  Port=2
  Add : Sum  AccumDataTypeStr=fixdt(1,16,0)
  Discrete FIR Filter HDL Optimized : dsphdlfiltering/Discrete FIR Filter HDL Optimized  Numerator=real(Taps)  Sharing=off  SharingFactor=2  SimulateUsing=Code generation  roundingMode=Floor  overflowMode=off  CoefficientsDataTypeStr=Inherit: Same word length as input  CoefficientsMin=[]  CoefficientsMax=[]  OutputDataTypeStr=fixdt(1,15,0)  OutputMin=[]  OutputMax=[]  ValidInPort=on  ReadyPort=off
      settings: SourceProductName=DSP System Toolbox  SourceProductBaseCode=DS
  Discrete FIR Filter HDL Optimized1 : dsphdlfiltering/Discrete FIR Filter HDL Optimized  Numerator=imag(Taps)  Sharing=off  SharingFactor=2  SimulateUsing=Code generation  roundingMode=Floor  overflowMode=off  CoefficientsDataTypeStr=Inherit: Same word length as input  CoefficientsMin=[]  CoefficientsMax=[]  OutputDataTypeStr=fixdt(1,15,0)  OutputMin=[]  OutputMax=[]  ValidInPort=on  ReadyPort=off
      settings: SourceProductName=DSP System Toolbox  SourceProductBaseCode=DS
  Logical Operator : Logic  AllPortsSameDT=off  OutDataTypeStr=boolean
  Out1 : Outport
  validOut : Outport  Port=2
  wires:
  In1/1 -> Discrete FIR Filter HDL Optimized1/1, Discrete FIR Filter HDL Optimized/1
  Discrete FIR Filter HDL Optimized/1 -> Add/1
  Add/1 -> Out1/1
  Logical Operator/1 -> validOut/1
  Discrete FIR Filter HDL Optimized/2 -> Logical Operator/1
  Discrete FIR Filter HDL Optimized1/2 -> Logical Operator/2
  Discrete FIR Filter HDL Optimized1/1 -> Add/2
  validIn/1 -> Discrete FIR Filter HDL Optimized1/2, Discrete FIR Filter HDL Optimized/2

== system RadioReceiver_FP_clean_PIPELINED/Receiver HDL/Frame Recover/Barker Locate/Measure Phase Ambiguity ==
  In1 : Inport  OutDataTypeStr=int16
  trigger : Inport  Port=2
  Discrete FIR Filter1 : DiscreteFir  Coefficients=exp(-j*pi/2).*xPreambleSeq(end:-1:1).'  AccumDataTypeStr=Inherit: Same as product output  OutDataTypeStr=int16
  Discrete FIR Filter2 : DiscreteFir  Coefficients=xPreambleSeq(end:-1:1).'  AccumDataTypeStr=Inherit: Same as product output  OutDataTypeStr=int16
  Discrete FIR Filter3 : DiscreteFir  Coefficients=exp(-j*pi).*xPreambleSeq(end:-1:1).'  AccumDataTypeStr=Inherit: Same as product output  OutDataTypeStr=int16
  Discrete FIR Filter4 : DiscreteFir  Coefficients=exp(-j*pi*3/2).*xPreambleSeq(end:-1:1).'  AccumDataTypeStr=Inherit: Same as product output  OutDataTypeStr=int16
  Find Max and Set Output Shift : Subsystem
  Out1 : Outport  InitialOutput=0
  wires:
  In1/1 -> Discrete FIR Filter4/1, Discrete FIR Filter3/1, Discrete FIR Filter1/1, Discrete FIR Filter2/1
  Discrete FIR Filter2/1 -> Find Max and Set Output Shift/1(In1)
  Discrete FIR Filter1/1 -> Find Max and Set Output Shift/2(In2)
  Discrete FIR Filter3/1 -> Find Max and Set Output Shift/3(In4)
  Discrete FIR Filter4/1 -> Find Max and Set Output Shift/4(In5)
  trigger/1 -> Find Max and Set Output Shift/Enable
  Find Max and Set Output Shift/1(Out1) -> Out1/1

== system RadioReceiver_FP_clean_PIPELINED/Receiver HDL/Frame Recover/Barker Locate/Measure Phase Ambiguity1 ==
  data : Inport  OutDataTypeStr=int16
  trigger : Inport  Port=2
  validIn : Inport  Port=3
  Find Max and Set Output Shift : Subsystem
  HDL Opt Complex FIR4 : Subsystem  mask{Taps=xPreambleSeq(end:-1:1).'}
  HDL Opt Complex FIR5 : Subsystem  mask{Taps=exp(-j*pi/2).*xPreambleSeq(end:-1:1).'}
  HDL Opt Complex FIR6 : Subsystem  mask{Taps=exp(-j*pi).*xPreambleSeq(end:-1:1).'}
  HDL Opt Complex FIR7 : Subsystem  mask{Taps=exp(-j*pi*3/2).*xPreambleSeq(end:-1:1).'}
  Logical Operator : Logic  Inputs=5  AllPortsSameDT=off  OutDataTypeStr=boolean
  PA : Outport  InitialOutput=0
  wires:
  data/1 -> HDL Opt Complex FIR4/1(In1), HDL Opt Complex FIR5/1(In1), HDL Opt Complex FIR7/1(In1), HDL Opt Complex FIR6/1(In1)
  HDL Opt Complex FIR4/1(Out1) -> Find Max and Set Output Shift/1(In1)
  HDL Opt Complex FIR5/1(Out1) -> Find Max and Set Output Shift/2(In2)
  HDL Opt Complex FIR6/1(Out1) -> Find Max and Set Output Shift/3(In4)
  HDL Opt Complex FIR7/1(Out1) -> Find Max and Set Output Shift/4(In5)
  Find Max and Set Output Shift/1(Out1) -> PA/1
  validIn/1 -> HDL Opt Complex FIR4/2(validIn), HDL Opt Complex FIR5/2(validIn), HDL Opt Complex FIR7/2(validIn), HDL Opt Complex FIR6/2(validIn)
  HDL Opt Complex FIR4/2(validOut) -> Logical Operator/1
  HDL Opt Complex FIR5/2(validOut) -> Logical Operator/2
  HDL Opt Complex FIR6/2(validOut) -> Logical Operator/3
  HDL Opt Complex FIR7/2(validOut) -> Logical Operator/4
  Logical Operator/1 -> Find Max and Set Output Shift/Enable
  trigger/1 -> Logical Operator/5

== system RadioReceiver_FP_clean_PIPELINED/Receiver HDL/Frame Recover/Equalization and Demodulation/2 Bit Descrambler ==
  note: This is a special Descrambler which can process 2 bits at a time
  u1 : Inport
  reset : Inport  Port=2
  Demux1 : Demux  Outputs=2
  MATLAB Function : MATLAB Function  TreatAsAtomicUnit=on
  Mux : Mux  Inputs=2
  Selector1 : Selector  IndexOptions=Index vector (dialog)  Indices=find(polynom(2:end))  OutputSizes=1
  Selector2 : Selector  IndexOptions=Index vector (dialog)  Indices=find(polynom(2:end))  OutputSizes=1
  input_xor1 : Logic  Operator=XOR  IconShape=distinctive  AllPortsSameDT=off  OutDataTypeStr=boolean
  input_xor2 : Logic  Operator=XOR  IconShape=distinctive  AllPortsSameDT=off  OutDataTypeStr=boolean
  state_xor1 : Logic  Operator=XOR  Inputs=1  IconShape=distinctive  AllPortsSameDT=off  OutDataTypeStr=boolean
  state_xor2 : Logic  Operator=XOR  Inputs=1  IconShape=distinctive  AllPortsSameDT=off  OutDataTypeStr=boolean
  y1 : Outport  InitialOutput=0
  wires:
  u1/1 -> Demux1/1, MATLAB Function/1(bits)
  reset/1 -> MATLAB Function/2(reset)
  MATLAB Function/1(bufferA) -> Selector1/1
  MATLAB Function/2(bufferB) -> Selector2/1
  Mux/1 -> y1/1
  state_xor1/1 -> input_xor1/1
  state_xor2/1 -> input_xor2/1
  input_xor2/1 -> Mux/2
  input_xor1/1 -> Mux/1
  Selector1/1 -> state_xor1/1
  Selector2/1 -> state_xor2/1
  Demux1/1 -> input_xor1/2
  Demux1/2 -> input_xor2/2  "data_in"

== system RadioReceiver_FP_clean_PIPELINED/Receiver HDL/Frame Recover/Equalization and Demodulation/DFE ==
  note: Generate training sequence when barker is found
  Trigger : Inport
  data : Inport  Port=2
  Delay data so DFE can reset : Delay  DelayLength=1
  Delay ref so DFE can reset : Delay  DelayLength=1
  Equalizer : MATLAB Function  TreatAsAtomicUnit=on
  PN Sequence Generator : commseqgen3/PN Sequence Generator  poly='z^5 + z^3 + z^1 + 1'  ini_sta=[1 1 1 0 0]  outBitMaskSource=Dialog parameter  shift=0  outVarSiz=off  maxOutSizeMode=Dialog parameter  maxOutSize=[10 1]  Ts=-1  sampPerFrame=1  reset=on  bitPackedOutputs=on  outDataType=Smallest unsigned integer  numPackedBits=2  bitPackDataSigned=off  bitPackedOutDType=Smallest integer
      settings: SourceProductName=Communications System Toolbox
  Packeted To Unpacked : Subsystem
  QPSK Modulator Baseband : commdigbbndpm3/QPSK Modulator Baseband  InType=Bit  Enc=Binary  Ph=pi/4  outDtype=Fixed-point  outWordLen=16  outUDDataType=sfix(16)  outFracLenMode=User-defined  outFracLen=14  outDataTypeStr=fixdt(1,16,14)  outLastDataTypeStr=fixdt(1,16,14)
  dataEQed : Outport
  wires:
  Trigger/1 -> Equalizer/1(trigger), PN Sequence Generator/1
  data/1 -> Delay data so DFE can reset/1
  PN Sequence Generator/1 -> Packeted To Unpacked/1(In1)
  Packeted To Unpacked/1(Out1) -> QPSK Modulator Baseband/1
  QPSK Modulator Baseband/1 -> Delay ref so DFE can reset/1
  Delay data so DFE can reset/1 -> Equalizer/2(data)
  Delay ref so DFE can reset/1 -> Equalizer/3(trainingSymbol)
  Equalizer/1(eqOut) -> dataEQed/1

== system RadioReceiver_FP_clean_PIPELINED/Receiver HDL/Frame Recover/Frequency Recovery/Loop Filter ==
  note: This inflation is necessary
  note: Proportional-plus-Integrator Loop Filter,
      | Infinite DC Response to guarantee convergence
  e : Inport
  Add1 : Sum  RndMeth=Nearest  OutDataTypeStr=Inherit: Same as first input
  Add2 : Sum  OutDataTypeStr=Inherit: Same as first input
  Data Type Conversion : DataTypeConversion  OutDataTypeStr=fixdt(1,25,20)
  Delay : Delay  DelayLength=1
  Delay3 : Delay  DelayLength=1
  Delay4 : Delay  DelayLength=1
  Flip Sign : MATLAB Function  Commented=on  TreatAsAtomicUnit=on
  Gain : Gain  Commented=on  Gain=-1.0  OutDataTypeStr=fixdt(1,25,20)
  K1 : Gain  Gain=K2  OutDataTypeStr=Inherit: Same as input
  K2 : Gain  Gain=K1  OutDataTypeStr=Inherit: Same as input
  Sum2 : Sum  OutDataTypeStr=Inherit: Same as first input
  v : Outport
  wires:
  K1/1 -> Sum2/1
  Add1/1 -> Sum2/2
  e/1 -> K2/1, K1/1
  K2/1 -> Delay/1, Add1/2
  Delay/1 -> Add1/1
  Sum2/1 -> Delay3/1
  Delay3/1 -> Add2/1
  Delay4/1 -> Add2/2
  Add2/1 -> Delay4/1, Flip Sign/1(u), Data Type Conversion/1, Gain/1
  Data Type Conversion/1 -> v/1

== system RadioReceiver_FP_clean_PIPELINED/Receiver HDL/Frame Recover/Frequency Recovery/PED For QPSK ==
  In1 : Inport
  Complex to Real-Imag1 : ComplexToRealImag
  Flip Sign : Subsystem
  Flip Sign1 : Subsystem
  Subtract1 : Sum  Inputs=+-
  Switch : Switch
  Switch1 : Switch
  Out1 : Outport
  wires:
  In1/1 -> Complex to Real-Imag1/1
  Complex to Real-Imag1/1 -> Flip Sign/1(In1), Switch1/1, Switch/2
  Complex to Real-Imag1/2 -> Flip Sign1/1(In1), Switch/1, Switch1/2
  Switch1/1 -> Subtract1/1
  Switch/1 -> Subtract1/2
  Flip Sign/1(Out1) -> Switch1/3
  Flip Sign1/1(Out1) -> Switch/3
  Subtract1/1 -> Out1/1

== system RadioReceiver_FP_clean_PIPELINED/Receiver HDL/Frame Recover/Frequency Recovery/PED For QPSK1 ==
  In1 : Inport
  Complex to Real-Imag : ComplexToRealImag
  Product : Product
  Product1 : Product
  Sign : Signum
  Sign1 : Signum
  Subtract : Sum  Inputs=+-
  Out1 : Outport
  wires:
  In1/1 -> Complex to Real-Imag/1
  Complex to Real-Imag/1 -> Product1/1, Sign/1
  Complex to Real-Imag/2 -> Product/2, Sign1/1
  Sign/1 -> Product/1
  Sign1/1 -> Product1/2
  Product/1 -> Subtract/1
  Product1/1 -> Subtract/2
  Subtract/1 -> Out1/1

== system RadioReceiver_FP_clean_PIPELINED/Receiver HDL/Frame Recover/Frequency Recovery/Phase Shift FP ==
  note: Sign Comes from original
      | loop filter design
  In1 : Inport
  Phi : Inport  Port=2
  Complex Phase Shift : commutil2/Complex Phase Shift  Commented=on
      settings: SourceProductName=Communications System Toolbox  SourceProductBaseCode=CM
  Cosine HDL Optimized : hdlsllib/Lookup Tables/Cosine HDL Optimized  OutputFormula=exp(j*2*pi*u)  NumDataPoints=256  TableDataTypeStr=fixdt(0,31,20)  SimulateLUTROMDelay=off
      settings: SourceProductName=HDL Coder  SourceProductBaseCode=HD
  Data Type Conversion1 : DataTypeConversion  Commented=on  OutDataTypeStr=double
  Data Type Conversion2 : DataTypeConversion  Commented=on  OutDataTypeStr=double
  Data Type Conversion3 : DataTypeConversion  Commented=on  OutDataTypeStr=fixdt(1,16,13)
  Gain : Gain  Gain=-1/(2*pi)  ParamDataTypeStr=fixdt(1,25,20)  OutDataTypeStr=fixdt(1,16,12)  SaturateOnIntegerOverflow=on
  Gain1 : Gain  Commented=on  Gain=-1/(2*pi)  ParamDataTypeStr=fixdt(1,25,20)  OutDataTypeStr=fixdt(1,25,20)  SaturateOnIntegerOverflow=on
  Product : Product  OutDataTypeStr=fixdt(1,16,13)  SaturateOnIntegerOverflow=on
  Out1 : Outport
  wires:
  Product/1 -> Out1/1
  Cosine HDL Optimized/1 -> Product/2
  In1/1 -> Data Type Conversion2/1, Product/1
  Phi/1 -> Data Type Conversion1/1, Gain/1
  Gain/1 -> Cosine HDL Optimized/1
  Complex Phase Shift/1 -> Data Type Conversion3/1
  Data Type Conversion2/1 -> Complex Phase Shift/1
  Data Type Conversion1/1 -> Complex Phase Shift/2

== system RadioReceiver_FP_clean_PIPELINED/Receiver HDL/Frame Recover/Gardner Reference/Gardner TED Blocks ==
  note: An input of 4 should not
      | happen unless the input is all zeros
  note: This is for QPSK and 4 SamplesPerSymbol ONLY
  data : Inport
  strobe : Inport  Port=2
  Add : Sum  OutDataTypeStr=fixdt(1,16,15)
  Check Only Strobe Condition : simulink/Logic and Bit Operations/Compare To Constant  relop===  const=uint8(1)  OutDataTypeStr=boolean
  Complex to Real-Imag : ComplexToRealImag
  Constant : Constant  Value=0  OutDataTypeStr=Inherit: Inherit via back propagation  SampleTime=-1
  Display : Display
  Imag Error : Subsystem
  Logical Operator : Logic  AllPortsSameDT=off  OutDataTypeStr=boolean
  Map [0,1,2,3,4] to [0,1,2,2,2] : LookupNDDirect  NumberOfTableDimensions=1  Table=[0 1 2 2 2]  DiagnosticForOutOfRangeInput=Error  TableDataTypeStr=uint8
  Real Error : Subsystem
  Strobe Buffer1 : simulink/Discrete/Tapped Delay  vinit=0.0  samptime=-1  NumDelays=samplesPerSymbol-1  DelayOrder=Oldest  includeCurrent=on
  Sum of Elements1 : Sum  Inputs=+  OutDataTypeStr=int8
  Switch : Switch  Criteria=u2 ~= 0  SaturateOnIntegerOverflow=on
  e : Outport
  wires:
  Switch/1 -> e/1
  strobe/1 -> Strobe Buffer1/1, Logical Operator/2
  Complex to Real-Imag/2 -> Imag Error/1(data)
  Sum of Elements1/1 -> Display/1, Check Only Strobe Condition/1, Map [0,1,2,3,4] to [0,1,2,2,2]/1
  Check Only Strobe Condition/1 -> Logical Operator/1
  Constant/1 -> Switch/3
  Complex to Real-Imag/1 -> Real Error/1(data)
  data/1 -> Complex to Real-Imag/1
  Map [0,1,2,3,4] to [0,1,2,2,2]/1 -> Imag Error/2(strobe sum), Real Error/2(strobe sum)
  Strobe Buffer1/1 -> Sum of Elements1/1
  Real Error/1(Out1) -> Add/1
  Imag Error/1(Out1) -> Add/2
  Add/1 -> Switch/1
  Logical Operator/1 -> Switch/2

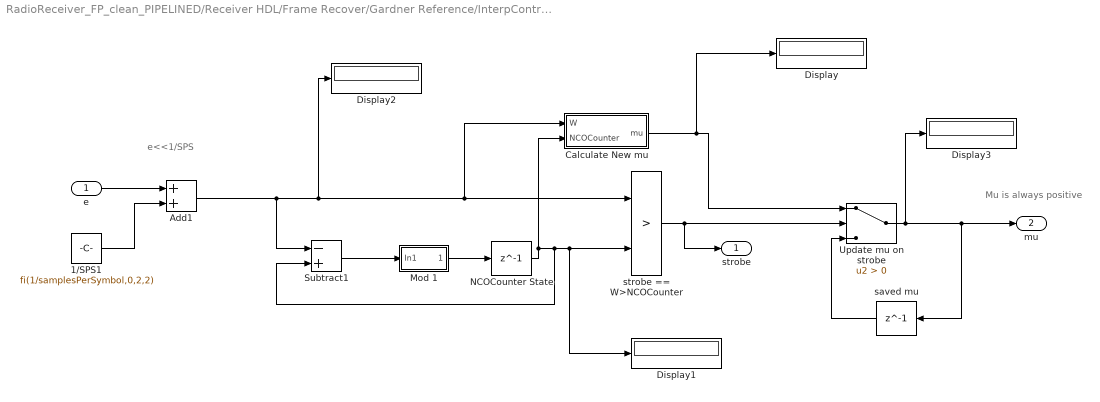
== system RadioReceiver_FP_clean_PIPELINED/Receiver HDL/Frame Recover/Gardner Reference/InterpControl_Blocks1 ==
  note: e<<1/SPS
  note: Mu is always positive
  e : Inport
  1/SPS1 : Constant  Value=fi(1/samplesPerSymbol,0,2,2)  OutDataTypeStr=fixdt(0,2,2)  SampleTime=-1
  Add1 : Sum  OutDataTypeStr=fixdt(0,16,16)
  Calculate New mu : Subsystem
  Display{,1..3} (4 alike) : Display
  Mod 1 : Subsystem
  NCOCounter State : Delay  DelayLength=1  InitialCondition=0
  Subtract1 : Sum  Inputs=-+  OutDataTypeStr=Inherit: Same as first input
  Update mu on strobe : Switch  Criteria=u2 > Threshold
  saved mu : Delay  DelayLength=1
  strobe == W>NCOCounter : RelationalOperator  Operator=>  OutDataTypeStr=boolean  RndMeth=Nearest
  strobe : Outport
  mu : Outport  Port=2
  wires:
  strobe == W>NCOCounter/1 -> Update mu on strobe/2, strobe/1
  Update mu on strobe/1 -> Display3/1, mu/1, saved mu/1
  saved mu/1 -> Update mu on strobe/3
  Calculate New mu/1(mu) -> Display/1, Update mu on strobe/1
  e/1 -> Add1/1
  NCOCounter State/1 -> Subtract1/2, Display1/1, strobe == W>NCOCounter/2, Calculate New mu/2(NCOCounter)
  Subtract1/1 -> Mod 1/1(In1)
  Mod 1/1(Out1) -> NCOCounter State/1
  1/SPS1/1 -> Add1/2
  Add1/1 -> Calculate New mu/1(W), strobe == W>NCOCounter/1, Display2/1, Subtract1/1

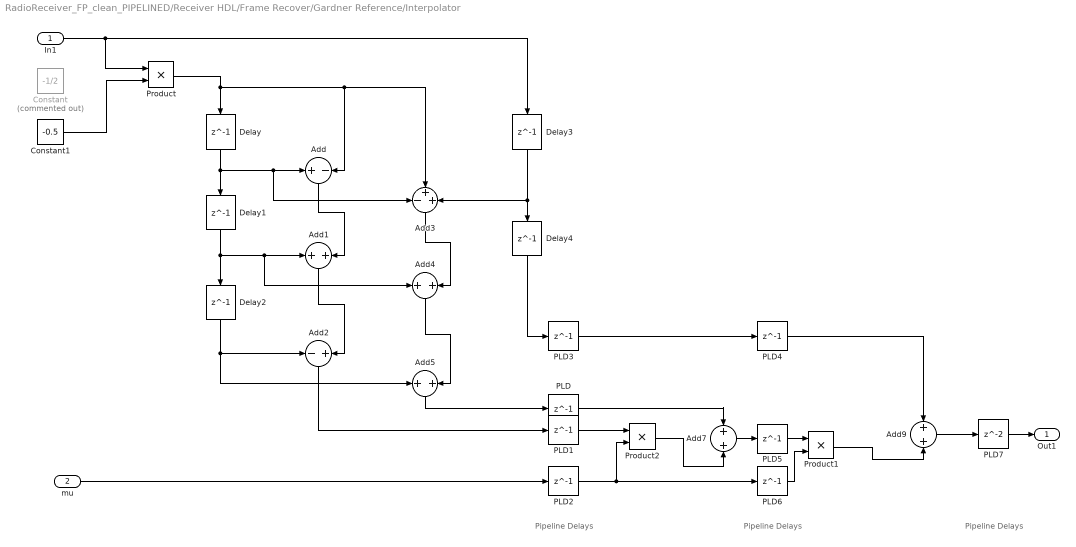
== system RadioReceiver_FP_clean_PIPELINED/Receiver HDL/Frame Recover/Gardner Reference/Interpolator ==
  note: Pipeline Delays
  note: Pipeline Delays
  note: Pipeline Delays
  In1 : Inport
  mu : Inport  Port=2
  Add : Sum  Inputs=+-  OutDataTypeStr=Inherit: Same as first input
  Add{1,4..5,7} (4 alike) : Sum
  Add2 : Sum  Inputs=-+
  Add3 : Sum  Inputs=-++
  Add9 : Sum  OutDataTypeStr=fixdt(1,16,10)
  Constant : Constant  Commented=on  Value=-1/2  OutDataTypeStr=double  SampleTime=-1
  Constant1 : Constant  Value=-0.5  OutDataTypeStr=fixdt(1,2,2)  SampleTime=-1
  Delay{,1..4} (5 alike) : Delay  DelayLength=1
  PLD{,1..6} (7 alike) : Delay  DelayLength=1
  PLD7 : Delay
  Product : Product  OutDataTypeStr=fixdt(1,16,14)
  Product1 : Product
  Product2 : Product  OutDataTypeStr=fixdt(1,16,10)
  Out1 : Outport
  wires:
  In1/1 -> Delay3/1, Product/1
  Product/1 -> Add3/2, Add/2, Delay/1
  Delay/1 -> Add3/1, Add/1, Delay1/1
  Delay1/1 -> Add4/1, Add1/1, Delay2/1
  Add/1 -> Add1/2
  Delay2/1 -> Add5/1, Add2/1
  Add1/1 -> Add2/2
  Add3/1 -> Add4/2
  Add4/1 -> Add5/2
  Add2/1 -> PLD1/1
  mu/1 -> PLD2/1
  Add5/1 -> PLD/1
  Product2/1 -> Add7/2
  Add9/1 -> PLD7/1
  Delay3/1 -> Delay4/1, Add3/3
  Delay4/1 -> PLD3/1
  Add7/1 -> PLD5/1
  Product1/1 -> Add9/2
  Constant1/1 -> Product/2
  PLD/1 -> Add7/1
  PLD1/1 -> Product2/1
  PLD2/1 -> Product2/2, PLD6/1
  PLD3/1 -> PLD4/1
  PLD4/1 -> Add9/1
  PLD5/1 -> Product1/1
  PLD6/1 -> Product1/2
  PLD7/1 -> Out1/1

== system RadioReceiver_FP_clean_PIPELINED/Receiver HDL/Frame Recover/Gardner Reference/LoopFilter1 ==
  e : Inport
  Delay1 : Delay  DelayLength=1
  Delay2 : Delay  DelayLength=1
  Proportional Gain : Gain  Gain=fi(ProportionalGain,1,16,15)  OutDataTypeStr=fixdt(1,16,24)
  v : Outport
  wires:
  e/1 -> Delay2/1
  Proportional Gain/1 -> Delay1/1
  Delay2/1 -> Proportional Gain/1
  Delay1/1 -> v/1

== system RadioReceiver_FP_clean_PIPELINED/Receiver HDL/Frame Recover/Barker Locate/Measure Phase Ambiguity/Find Max and Set Output Shift ==
  In1 : Inport  OutDataTypeStr=int16
  In2 : Inport  Port=2  OutDataTypeStr=int16
  In4 : Inport  Port=3  OutDataTypeStr=int16
  In5 : Inport  Port=4  OutDataTypeStr=int16
  Enable : EnablePort
  Complex to Real-Imag{,1..3} (4 alike) : ComplexToRealImag  Output=Imag
  Direct Lookup Table (n-D) : LookupNDDirect  NumberOfTableDimensions=1  Table=exp(-(0:pi/2:(pi*3/2)) .* 1i).'  DiagnosticForOutOfRangeInput=Error  TableDataTypeStr=fixdt(1,16,13)
  Maximum : dspstat3/Maximum  operation=maximum  fcn=Index  indexBase=Zero  operateOver=Each column  Dimension=1  InputProcessing=Columns as channels (frame based)  reset=None  roiEnable=off  roiType=Rectangles  roiPortion=Entire ROI  roiOutput=Individual statistics for each ROI  roiFlag=off  roundingMode=Floor  overflowMode=off  accumDataTypeStr=Inherit: Same as product output  accumLastDataTypeStr=Inherit: Same as product output
  Vector Concatenate : Concatenate  NumInputs=4
  Out1 : Outport  InitialOutput=0
  wires:
  Direct Lookup Table (n-D)/1 -> Out1/1
  In1/1 -> Complex to Real-Imag/1
  Complex to Real-Imag2/1 -> Vector Concatenate/3
  Complex to Real-Imag1/1 -> Vector Concatenate/2
  In5/1 -> Complex to Real-Imag3/1
  Complex to Real-Imag3/1 -> Vector Concatenate/4
  Complex to Real-Imag/1 -> Vector Concatenate/1
  Maximum/1 -> Direct Lookup Table (n-D)/1
  In2/1 -> Complex to Real-Imag1/1
  Vector Concatenate/1 -> Maximum/1
  In4/1 -> Complex to Real-Imag2/1

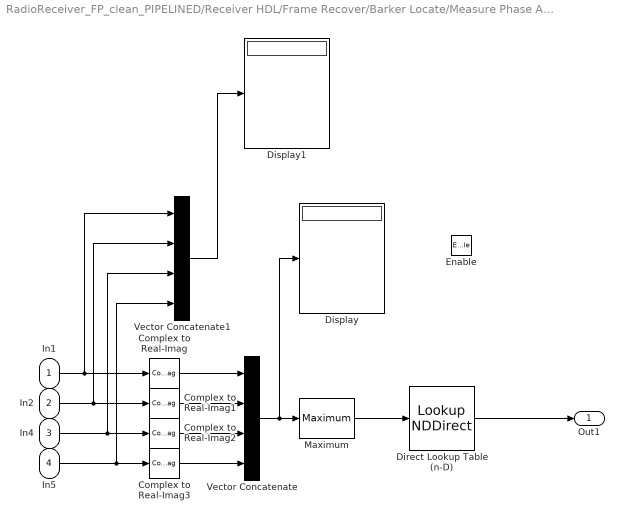
== system RadioReceiver_FP_clean_PIPELINED/Receiver HDL/Frame Recover/Barker Locate/Measure Phase Ambiguity1/Find Max and Set Output Shift ==
  In1 : Inport
  In2 : Inport  Port=2
  In4 : Inport  Port=3
  In5 : Inport  Port=4
  Enable : EnablePort
  Complex to Real-Imag{,1..3} (4 alike) : ComplexToRealImag  Output=Imag
  Direct Lookup Table (n-D) : LookupNDDirect  NumberOfTableDimensions=1  Table=exp(-(0:pi/2:(pi*3/2)) .* 1i).'  DiagnosticForOutOfRangeInput=Error  TableDataTypeStr=fixdt(1,16,13)
  Display : Display
  Display1 : Display
  Maximum : dspstat3/Maximum  operation=maximum  fcn=Index  indexBase=Zero  operateOver=Each column  Dimension=1  InputProcessing=Columns as channels (frame based)  reset=None  roiEnable=off  roiType=Rectangles  roiPortion=Entire ROI  roiOutput=Individual statistics for each ROI  roiFlag=off  roundingMode=Floor  overflowMode=off  accumDataTypeStr=Inherit: Same as product output  accumLastDataTypeStr=Inherit: Same as product output
  Vector Concatenate : Concatenate  NumInputs=4
  Vector Concatenate1 : Concatenate  NumInputs=4
  Out1 : Outport  InitialOutput=0
  wires:
  Direct Lookup Table (n-D)/1 -> Out1/1
  In4/1 -> Vector Concatenate1/3, Complex to Real-Imag2/1
  In2/1 -> Vector Concatenate1/2, Complex to Real-Imag1/1
  In5/1 -> Vector Concatenate1/4, Complex to Real-Imag3/1
  In1/1 -> Vector Concatenate1/1, Complex to Real-Imag/1
  Maximum/1 -> Direct Lookup Table (n-D)/1
  Vector Concatenate/1 -> Display/1, Maximum/1
  Vector Concatenate1/1 -> Display1/1
  Complex to Real-Imag1/1 -> Vector Concatenate/2
  Complex to Real-Imag3/1 -> Vector Concatenate/4
  Complex to Real-Imag2/1 -> Vector Concatenate/3
  Complex to Real-Imag/1 -> Vector Concatenate/1
